simulink model "modelo_termico"  (R2019b)
settings: Solver=VariableStepAuto  StartTime=0.0  StopTime=10.0  RelTol=1e-3
values from neighbouring files (symbols this model uses):
  k = [0 1 2 3 4 5 6 7 8 9 10 11 ... (20000 elements, 1x20000)]    [butter1.mat]    (also in media_movel_geral.mat = [0 1 2 3 4 5 6 7 8 9 10 11 ... (51 elements, 1x51)]; modelo_termico.mat = 0.01)
  T = 0.00833333333333    [ECG_graficos_fft.mat]    (also in FPB_Arduino.mat = 0.001; butter1.mat = 1.25e-08; filtro_notch1.mat; intro_resp_freq.mat = 0.00125)
settings Model: Creator=fernandopassold  LastModifiedBy=fernandopassold

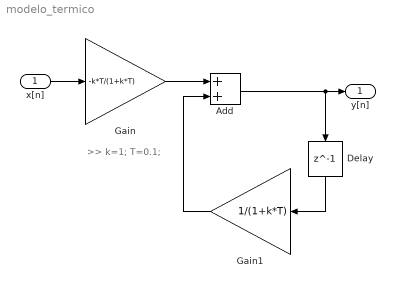
== system modelo_termico ==
  note: >> k=1; T=0.1;
  x[n] : Inport
  Add : Sum
  Delay : Delay  DelayLength=1
  Gain : Gain  Gain=-k*T/(1+k*T)
  Gain1 : Gain  Gain=1/(1+k*T)
  y[n] : Outport
  wires:
  x[n]/1 -> Gain/1
  Gain/1 -> Add/1
  Add/1 -> Delay/1, y[n]/1
  Delay/1 -> Gain1/1
  Gain1/1 -> Add/2
